simulink model "no3_PI_Controller"  (R2025a)
settings: Solver=VariableStepAuto  StartTime=0.0  StopTime=50  RelTol=1e-3
libraries: simulink x1
settings Model: Creator=ayeo  LastModifiedBy=ayeo

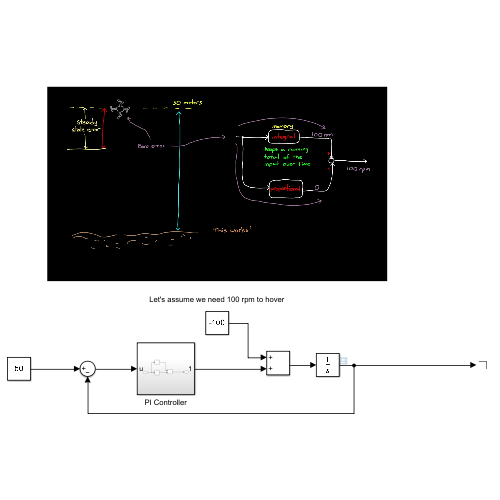
[thumbnail: Simulink's stored preview of the top-level diagram]
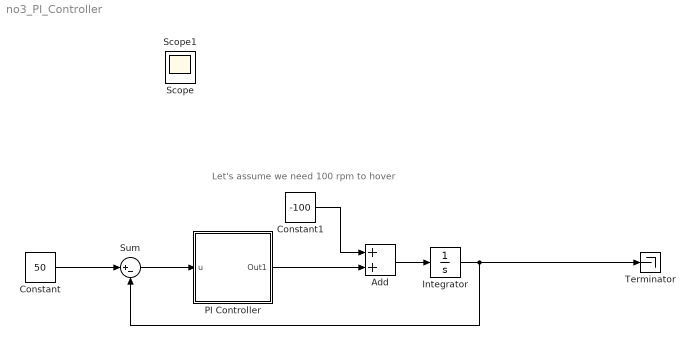
== system no3_PI_Controller ==
  note: Let's assume we need 100 rpm to hover
  Add : Sum
  Constant : Constant  Value=50
  Constant1 : Constant  Value=-100
  Integrator : Integrator
  PI Controller : Subsystem
  Sum : Sum  Inputs=|+-
  Terminator : Terminator
  Scope : Scope
      settings: ActiveDisplayYMinimum=-74.47126  ActiveDisplayYMaximum=162.49353
  Scope1 : Scope
      settings: ActiveDisplayYMinimum=81.26535  ActiveDisplayYMaximum=268.74829
  wires:
  Constant/1 -> Sum/1
  Integrator/1 -> Sum/2, Terminator/1
  Add/1 -> Integrator/1
  Constant1/1 -> Add/1
  Sum/1 -> PI Controller/1(u)
  PI Controller/1(Out1) -> Add/2

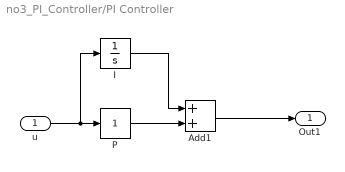
== system no3_PI_Controller/PI Controller ==
  u : Inport
  Add1 : Sum
  I : Integrator
  P : simulink/Math Operations/Slider Gain  gain=1  low=0.1  high=100
  Out1 : Outport
  wires:
  P/1 -> Add1/2
  u/1 -> I/1, P/1
  Add1/1 -> Out1/1
  I/1 -> Add1/1
